simulink model "scd3busMicrogridDroopControlFidelityLevels2Inv"  (R2025b)
settings: Solver=ode15s  StartTime=0.0  StopTime=24  RelTol=1e-3
PreLoadFcn:
  | scd3busMicrogridDroopControlDataFidelityLevels2Inv;
  | 
  | %% Controller variants
  | % Create variant controls for converter controller. Controller has two
  | % different levels of fidelity: Averaged, AveragedPulse, Pulse
  | Averaged = Simulink.VariantExpression;
  | Averaged.Condition = 'fidelity==scd3busMicrogridDroopControl_variants_enum.Low';
  | Pulse = Simulink.VariantExpression;
  | Pulse.Condition = 'fidelity==scd3busMicrogridDroopControl_variants_enum.High';
  | 
  | %% Plant variants
  | % Create variant controls for converter plant. Plant has three different
  | % levels of fidelity.
  | AveragedNonSwitch = Simulink.VariantExpression;
  | AveragedNonSwitch.Condition = 'fidelity==scd3busMicrogridDroopControl_variants_enum.Low';
  | PulseSwitch = Simulink.VariantExpression;
  | PulseSwitch.Condition = 'fidelity==scd3busMicrogridDroopControl_variants_enum.High';
  | 
  | %% Set up variables ready for simulation
  | fidelity = scd3busMicrogridDroopControl_variants_enum.High;
  | Ts = 5e-6;
  | Ts_V = 1e-6;
  | Tsc = 1e-4;
  | Tsc_V = 5e-4;
values from neighbouring files (symbols this model uses):
  consensus_enable = 1    [scd3busMicrogridDroopControlDataFidelityLevels3Inv.m]
  fgrid = 60    [scd3busMicrogridDroopControlDataFidelityLevels.m]    (also in scd3busMicrogridDroopControlDataFidelityLevels3Inv.m)
  Kdroop_fp1 = 0.03/2    (= 0.015)    [scd3busMicrogridDroopControlDataFidelityLevels3Inv.m]
  Kdroop_fp2 = 0.03/2    (= 0.015)    [scd3busMicrogridDroopControlDataFidelityLevels3Inv.m]
  Kdroop_vq1 = 0.05/2    (= 0.025)    [scd3busMicrogridDroopControlDataFidelityLevels3Inv.m]
  Kdroop_vq2 = 0.05/2    (= 0.025)    [scd3busMicrogridDroopControlDataFidelityLevels3Inv.m]
  Ki_vd = 850    [scd3busMicrogridDroopControlDataFidelityLevels.m]    (also in scd3busMicrogridDroopControlDataFidelityLevels3Inv.m)
  Ki_vq = 850    [scd3busMicrogridDroopControlDataFidelityLevels.m]    (also in scd3busMicrogridDroopControlDataFidelityLevels3Inv.m)
  Kp_vd = 0.36    [scd3busMicrogridDroopControlDataFidelityLevels.m]    (also in scd3busMicrogridDroopControlDataFidelityLevels3Inv.m)
  Kp_vq = 0.36    [scd3busMicrogridDroopControlDataFidelityLevels.m]    (also in scd3busMicrogridDroopControlDataFidelityLevels3Inv.m)
  Vdc1 = 1000    [scd3busMicrogridDroopControlDataFidelityLevels.m]    (also in scd3busMicrogridDroopControlDataFidelityLevels3Inv.m)
  Vdc2 = 1000    [scd3busMicrogridDroopControlDataFidelityLevels.m]    (also in scd3busMicrogridDroopControlDataFidelityLevels3Inv.m)
  Vrms = 380    [scd3busMicrogridDroopControlDataFidelityLevels.m]    (also in scd3busMicrogridDroopControlDataFidelityLevels3Inv.m)
undefined symbols (not defined in the file or in its folder): DiscIntNeverNeededParam
libraries: ee_lib x29, nesl_utility x29, fl_lib x17, eeTransforms x4, eeSinusoidalMeasurement x4, slpidlib x4, eePwmGeneratorTwoLevel x2, eePowerMeasurement x2, simulink x2, SignalEditorBlockLib x1
(part 3 of 3)

== system scd3busMicrogridDroopControlFidelityLevels2Inv/Inverter 2/Averaged Inverter ==
  Averaged Inverter : ee_lib/Semiconductors & Converters/Converters/Converter (Three-Phase)  port_option=ee.enum.threePhasePort.expanded  fidelity_option=ee.enum.converters.fidelity.detailed  device_type=ee.enum.converters.switchingdevice.averaged  showThermalPort=false  K=0  Vth=0.5 V  Vgt=1e-3 V  Vgt_off=-1 V  Ih=1 A  Vf=0.8 V  Ron=1.0000e-03 Ohm  Rds=0.001 Ohm  Goff=2.0000e-04 1/Ohm  Eon_scalar=22.86e-3 J  Eoff_scalar=17.14e-3 J  Eoff_natural_commutation=10e-3 J  Voff=300 V  Iout_scalar=600 A  onCurrentMeasDelay=0 s  useCurrentFromPreviousCycle=false  useVoltageFromPreviousCycle=false  diode_param=ee.enum.converters.protectiondiode.nodynamics  diode_Vf=0.8 V  diode_Ron=0.001 Ohm  diode_Goff=1e-5 1/Ohm  diode_C=50 nF  diode_iRM=-235 A  diode_iF=300 A  diode_idot=-50 A/us  diode_trr_param=ee.enum.converters.diodetrr.trr_factor  diode_trr_factor=3  diode_trr=15 us  diode_Qrr=1.5e+3 s*uA  diode_rec_loss_model=ee.enum.diode.reverseRecoveryModel.fixed  diode_ErecVal=0 J  diode_scaleWithIandV=false  diode_ErecMat=zeros(2, 3) J  diode_TjrecVec=[298.15, 398.15] K  diode_IfrecVec=[.1, 1, 10] A  diode_IrecVal=10 A  diode_VrecVal=10 V  diode_tFilter=1 / 1000 / 100 s  thermal_network_parameterization=ee.enum.thermalNetworkTopology.external  Rth=[.08, .5] K/W  Rth_Cauer=[.08, .1, .5] K/W  Rth_Foster=[.08, .14, .22, .16] K/W  thermal_mass_parameterization=ee.enum.thermalNetwork.timeconstant  thermal_mass=[.01, .5] J/K  thermal_mass_Cauer=[.01, .1, .5] J/K  thermal_mass_Foster=[.001, .005, .05, .5] J/K  thermal_time_constant=[.001, .2] s  thermal_time_constant_Cauer=[.001, .1, .2] s  thermal_time_constant_Foster=[7e-05, .0007, .01, .08] s  thermal_mass_initial_temperatures=[25, 25] degC  thermal_mass_initial_temperatures_Cauer=[25, 25, 25] degC  junction_thermal_mass=0.01 J/K  Tvec_initial_Foster=[25, 25, 25, 25] degC  snubber_type=ee.enum.converters.snubber.exclude  Cs=1e-7 F  Rs=0.1 Ohm  Vce_loss=[0, 150, 300] V
      settings: InternalSimscapePortConfiguration="{\"Bottom\":[],\"Left\":[{\"id\":\"G\",\"label\":\"G\",\"type\":\"foundation.electrical.twelve_phase\"},{\"id\":\"a\",\"label\":\"a\",\"type\":\"foundation.electrical.electrical\"},{\"id\":\"b\",\"label\":\"b\",\"type\":\"foundation.electrical.electrical\"},{\"id\":\"c\",\"label\":\"c\",\"type\":\"foundation.electrical.electrical\"}],\"Right\":[{\"id\":\"p\",\"label\":\"+\",\"type\":\"foundation.electrical.electrical\"},{\"id\":\"n\",\"label\":\"-\",\"type\":\"foundation.electrical.electrical\"}],\"Top\":[]}"
  + : PMIOPort  Side=Right
  G : PMIOPort  Port=2  Side=Left
  a : PMIOPort  Port=3  Side=Left
  b : PMIOPort  Port=4  Side=Left
  - : PMIOPort  Port=5  Side=Right
  c : PMIOPort  Port=6  Side=Left
  connections:
  +/RConn1 -- Averaged Inverter/RConn1
  b/RConn1 -- Averaged Inverter/LConn3
  -/RConn1 -- Averaged Inverter/RConn2
  G/RConn1 -- Averaged Inverter/LConn1
  a/RConn1 -- Averaged Inverter/LConn2
  c/RConn1 -- Averaged Inverter/LConn4

== system scd3busMicrogridDroopControlFidelityLevels2Inv/Inverter 2/IGBT Inverter ==
  IGBT Inverter : ee_lib/Semiconductors & Converters/Converters/Converter (Three-Phase)  port_option=ee.enum.threePhasePort.expanded  fidelity_option=ee.enum.converters.fidelity.detailed  device_type=ee.enum.converters.switchingdevice.igbt  showThermalPort=false  K=0  Vth=0.5 V  Vgt=1e-3 V  Vgt_off=-1 V  Ih=1 A  Vf=0.8 V  Ron=1.0000e-03 Ohm  Rds=0.001 Ohm  Goff=2.0000e-04 1/Ohm  Eon_scalar=22.86e-3 J  Eoff_scalar=17.14e-3 J  Eoff_natural_commutation=10e-3 J  Voff=300 V  Iout_scalar=600 A  onCurrentMeasDelay=0 s  useCurrentFromPreviousCycle=false  useVoltageFromPreviousCycle=false  diode_param=ee.enum.converters.protectiondiode.nodynamics  diode_Vf=0.8 V  diode_Ron=0.001 Ohm  diode_Goff=1e-5 1/Ohm  diode_C=50 nF  diode_iRM=-235 A  diode_iF=300 A  diode_idot=-50 A/us  diode_trr_param=ee.enum.converters.diodetrr.trr_factor  diode_trr_factor=3  diode_trr=15 us  diode_Qrr=1.5e+3 s*uA  diode_rec_loss_model=ee.enum.diode.reverseRecoveryModel.fixed  diode_ErecVal=0 J  diode_scaleWithIandV=false  diode_ErecMat=zeros(2, 3) J  diode_TjrecVec=[298.15, 398.15] K  diode_IfrecVec=[.1, 1, 10] A  diode_IrecVal=10 A  diode_VrecVal=10 V  diode_tFilter=1 / 1000 / 100 s  thermal_network_parameterization=ee.enum.thermalNetworkTopology.external  Rth=[.08, .5] K/W  Rth_Cauer=[.08, .1, .5] K/W  Rth_Foster=[.08, .14, .22, .16] K/W  thermal_mass_parameterization=ee.enum.thermalNetwork.timeconstant  thermal_mass=[.01, .5] J/K  thermal_mass_Cauer=[.01, .1, .5] J/K  thermal_mass_Foster=[.001, .005, .05, .5] J/K  thermal_time_constant=[.001, .2] s  thermal_time_constant_Cauer=[.001, .1, .2] s  thermal_time_constant_Foster=[7e-05, .0007, .01, .08] s  thermal_mass_initial_temperatures=[25, 25] degC  thermal_mass_initial_temperatures_Cauer=[25, 25, 25] degC  junction_thermal_mass=0.01 J/K  Tvec_initial_Foster=[25, 25, 25, 25] degC  snubber_type=ee.enum.converters.snubber.exclude  Cs=1e-7 F  Rs=0.1 Ohm  Vce_loss=[0, 150, 300] V
      settings: InternalSimscapePortConfiguration="{\"Bottom\":[],\"Left\":[{\"id\":\"G\",\"label\":\"G\",\"type\":\"foundation.electrical.twelve_phase\"},{\"id\":\"a\",\"label\":\"a\",\"type\":\"foundation.electrical.electrical\"},{\"id\":\"b\",\"label\":\"b\",\"type\":\"foundation.electrical.electrical\"},{\"id\":\"c\",\"label\":\"c\",\"type\":\"foundation.electrical.electrical\"}],\"Right\":[{\"id\":\"p\",\"label\":\"+\",\"type\":\"foundation.electrical.electrical\"},{\"id\":\"n\",\"label\":\"-\",\"type\":\"foundation.electrical.electrical\"}],\"Top\":[]}"
  + : PMIOPort  Side=Right
  G : PMIOPort  Port=2  Side=Left
  a : PMIOPort  Port=3  Side=Left
  b : PMIOPort  Port=4  Side=Left
  - : PMIOPort  Port=5  Side=Right
  c : PMIOPort  Port=6  Side=Left
  connections:
  c/RConn1 -- IGBT Inverter/LConn4
  a/RConn1 -- IGBT Inverter/LConn2
  G/RConn1 -- IGBT Inverter/LConn1
  -/RConn1 -- IGBT Inverter/RConn2
  b/RConn1 -- IGBT Inverter/LConn3
  +/RConn1 -- IGBT Inverter/RConn1

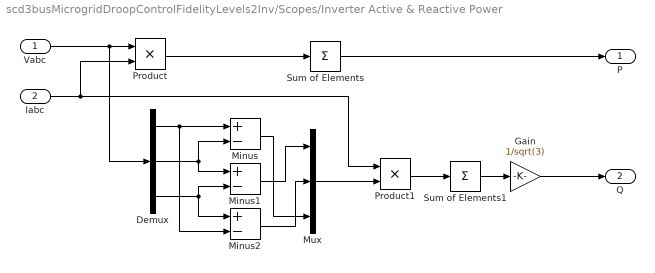
== system scd3busMicrogridDroopControlFidelityLevels2Inv/Scopes/Inverter Active & Reactive Power  ==
  Vabc : Inport
  Iabc : Inport  Port=2
  Demux : Demux  Outputs=3
  Gain : Gain  Gain=1/sqrt(3)
  Minus : Sum  Inputs=+-
  Minus1 : Sum  Inputs=+-
  Minus2 : Sum  Inputs=+-
  Mux : Mux  Inputs=3
  Product : Product
  Product1 : Product
  Sum of Elements : Sum  Inputs=+
  Sum of Elements1 : Sum  Inputs=+
  P : Outport  VectorParamsAs1DForOutWhenUnconnected=off
  Q : Outport  Port=2  VectorParamsAs1DForOutWhenUnconnected=off
  wires:
  Minus/1 -> Mux/3
  Minus2/1 -> Mux/2
  Minus1/1 -> Mux/1
  Gain/1 -> Q/1
  Sum of Elements1/1 -> Gain/1
  Product1/1 -> Sum of Elements1/1
  Mux/1 -> Product1/2
  Demux/3 -> Minus1/2, Minus2/1
  Demux/2 -> Minus/2, Minus1/1
  Demux/1 -> Minus/1, Minus2/2
  Sum of Elements/1 -> P/1
  Product/1 -> Sum of Elements/1
  Iabc/1 -> Product/2, Product1/1
  Vabc/1 -> Product/1, Demux/1

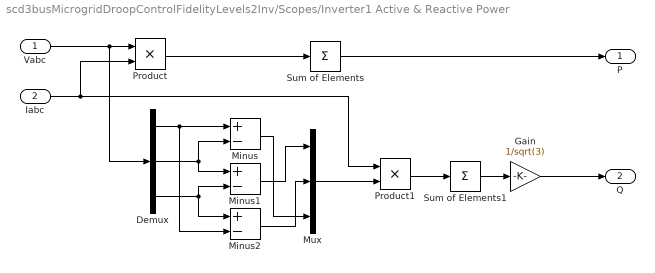
== system scd3busMicrogridDroopControlFidelityLevels2Inv/Scopes/Inverter1 Active & Reactive Power ==
  Vabc : Inport
  Iabc : Inport  Port=2
  Demux : Demux  Outputs=3
  Gain : Gain  Gain=1/sqrt(3)
  Minus : Sum  Inputs=+-
  Minus1 : Sum  Inputs=+-
  Minus2 : Sum  Inputs=+-
  Mux : Mux  Inputs=3
  Product : Product
  Product1 : Product
  Sum of Elements : Sum  Inputs=+
  Sum of Elements1 : Sum  Inputs=+
  P : Outport  VectorParamsAs1DForOutWhenUnconnected=off
  Q : Outport  Port=2  VectorParamsAs1DForOutWhenUnconnected=off
  wires:
  Vabc/1 -> Demux/1, Product/1
  Iabc/1 -> Product1/1, Product/2
  Product/1 -> Sum of Elements/1
  Sum of Elements/1 -> P/1
  Demux/1 -> Minus2/2, Minus/1
  Demux/2 -> Minus1/1, Minus/2
  Demux/3 -> Minus2/1, Minus1/2
  Mux/1 -> Product1/2
  Product1/1 -> Sum of Elements1/1
  Sum of Elements1/1 -> Gain/1
  Gain/1 -> Q/1
  Minus1/1 -> Mux/1
  Minus2/1 -> Mux/2
  Minus/1 -> Mux/3

== system scd3busMicrogridDroopControlFidelityLevels2Inv/Solar1/MPPT Algorithm ==
  I : Inport
  V : Inport  Port=2
  D_init : Constant  Value=0.25
  D_max : Constant  Value=0.4
  D_min : Constant  Value=0.15
  Delta_D : Constant  Value=0.001
  MPPT Algorithm : MATLAB Function  SystemSampleTime=Ts
  Unit Delay : UnitDelay  InitialCondition=0.2  SampleTime=0.01
  Vector Concatenate : Concatenate  NumInputs=4
  duty_cycle : Outport
  wires:
  V/1 -> MPPT Algorithm/2(V)
  Vector Concatenate/1 -> MPPT Algorithm/1(Param)
  D_max/1 -> Vector Concatenate/2
  D_init/1 -> Vector Concatenate/1
  D_min/1 -> Vector Concatenate/3
  MPPT Algorithm/1(D) -> Unit Delay/1
  Delta_D/1 -> Vector Concatenate/4
  I/1 -> MPPT Algorithm/3(I)
  Unit Delay/1 -> duty_cycle/1

== system scd3busMicrogridDroopControlFidelityLevels2Inv/Solar1/Sensing Current ==
  Current Sensor : fl_lib/Electrical/Electrical Sensors/Current Sensor
  PS-Simulink/I : nesl_utility/PS-Simulink Converter  PhysicalDomain=network_engine_domain  SubClassName=ps_output  LeftPortType=input  RightPortType=output  PseudoPeriodic=off  Frequencies=[]  VectorFormat=1-D array  Unit=1  AffineConversion=off
  + : PMIOPort  Side=Left
  - : PMIOPort  Port=2  Side=Right
  I : Outport
  wires:
  PS-Simulink/I/1 -> I/1
  connections:
  -/RConn1 -- Current Sensor/RConn2
  Current Sensor/LConn1 -- +/RConn1
  Current Sensor/RConn1 -- PS-Simulink/I/LConn1

== system scd3busMicrogridDroopControlFidelityLevels2Inv/Solar1/sensing voltage ==
  PS-Simulink Converter : nesl_utility/PS-Simulink Converter  PhysicalDomain=network_engine_domain  SubClassName=ps_output  LeftPortType=input  RightPortType=output  PseudoPeriodic=off  Frequencies=[]  VectorFormat=1-D array  Unit=inherit  AffineConversion=off
  Voltage Sensor : fl_lib/Electrical/Electrical Sensors/Voltage Sensor
  + : PMIOPort  Side=Left
  - : PMIOPort  Port=2  Side=Right
  V : Outport
  wires:
  PS-Simulink Converter/1 -> V/1
  connections:
  Voltage Sensor/LConn1 -- +/RConn1
  Voltage Sensor/RConn2 -- -/RConn1
  Voltage Sensor/RConn1 -- PS-Simulink Converter/LConn1

== system scd3busMicrogridDroopControlFidelityLevels2Inv/Solar2/MPPT Algorithm ==
  I : Inport
  V : Inport  Port=2
  D_init : Constant  Value=0.25
  D_max : Constant  Value=0.4
  D_min : Constant  Value=0.15
  Delta_D : Constant  Value=0.001
  MPPT Algorithm : MATLAB Function  SystemSampleTime=Ts
  Unit Delay : UnitDelay  InitialCondition=0.2  SampleTime=0.01
  Vector Concatenate : Concatenate  NumInputs=4
  duty_cycle : Outport
  wires:
  V/1 -> MPPT Algorithm/2(V)
  Vector Concatenate/1 -> MPPT Algorithm/1(Param)
  D_max/1 -> Vector Concatenate/2
  D_init/1 -> Vector Concatenate/1
  D_min/1 -> Vector Concatenate/3
  MPPT Algorithm/1(D) -> Unit Delay/1
  Delta_D/1 -> Vector Concatenate/4
  I/1 -> MPPT Algorithm/3(I)
  Unit Delay/1 -> duty_cycle/1

== system scd3busMicrogridDroopControlFidelityLevels2Inv/Solar2/Sensing Current ==
  Current Sensor : fl_lib/Electrical/Electrical Sensors/Current Sensor
  PS-Simulink/I : nesl_utility/PS-Simulink Converter  PhysicalDomain=network_engine_domain  SubClassName=ps_output  LeftPortType=input  RightPortType=output  PseudoPeriodic=off  Frequencies=[]  VectorFormat=1-D array  Unit=1  AffineConversion=off
  + : PMIOPort  Side=Left
  - : PMIOPort  Port=2  Side=Right
  I : Outport
  wires:
  PS-Simulink/I/1 -> I/1
  connections:
  -/RConn1 -- Current Sensor/RConn2
  Current Sensor/LConn1 -- +/RConn1
  Current Sensor/RConn1 -- PS-Simulink/I/LConn1

== system scd3busMicrogridDroopControlFidelityLevels2Inv/Solar2/sensing voltage ==
  PS-Simulink Converter : nesl_utility/PS-Simulink Converter  PhysicalDomain=network_engine_domain  SubClassName=ps_output  LeftPortType=input  RightPortType=output  PseudoPeriodic=off  Frequencies=[]  VectorFormat=1-D array  Unit=inherit  AffineConversion=off
  Voltage Sensor : fl_lib/Electrical/Electrical Sensors/Voltage Sensor
  + : PMIOPort  Side=Left
  - : PMIOPort  Port=2  Side=Right
  V : Outport
  wires:
  PS-Simulink Converter/1 -> V/1
  connections:
  Voltage Sensor/LConn1 -- +/RConn1
  Voltage Sensor/RConn2 -- -/RConn1
  Voltage Sensor/RConn1 -- PS-Simulink Converter/LConn1

== matlab function scd3busMicrogridDroopControlFidelityLevels2Inv/Solar1/MPPT Algorithm/MPPT Algorithm ==
  settings: updateMethod=DISCRETE  sampleTime=Ts_DC
  data: Param input; V input; I input; D output
function D = PandO(Param, V, I)

Dinit  = Param(1);
Dmax   = Param(2);
Dmin   = Param(3);
deltaD = Param(4);

persistent Vold Pold Dold;
if isempty(Vold)
    Vold = 0;
    Pold = 0;
    Dold = Dinit;
end

P  = V * I;
dV = V - Vold;
dP = P - Pold;

%% -- fixed: use a dead-band instead of exact zero comparison --
if abs(dP) < 0.5        % ignore changes smaller than 0.5 W (noise)
    D = Dold;           % already at MPP, hold duty cycle

elseif dP < 0
    if dV < 0
        D = Dold - deltaD;
    else
        D = Dold + deltaD;
    end

else                    % dP > 0
    if dV < 0
        D = Dold + deltaD;
    else
        D = Dold - deltaD;
    end
end

%% -- clamp --
D = max(Dmin, min(Dmax, D));

%% -- update persistent state --
Dold = D;
Vold = V;
Pold = P;

== matlab function scd3busMicrogridDroopControlFidelityLevels2Inv/Droop Controller Inverter1/MATLAB Function ==
  data: omega_1 input; d_omega output; omega_2 input; V_1 input; V_2 input; int_w_in input; int_v_in input; Ts input; d_V output; int_w_out output; int_v_out output
function [d_omega, d_V, int_w_out, int_v_out] = ...
         Consensus_Agent1(omega_1, omega_2, V_1, V_2, ...
                          int_w_in, int_v_in, Ts)
%% Gains — tuned for Hz units and visible correction
alpha_w = 50.0;   beta_w = 30.0;   kref_w = 20.0;
alpha_v = 0.30;   beta_v = 0.20;   kref_v = 0.10;

omega_ref = 60.0;   % Hz — confirmed from your freq_mea display
V_ref     = 1.0;    % pu

%% Frequency
e_omega     = omega_1 - omega_ref;
consensus_w = omega_1 - omega_2;
int_w_out   = max(-0.5, min(0.5, int_w_in + Ts * consensus_w));
d_omega     = -alpha_w*consensus_w - beta_w*int_w_out - kref_w*e_omega;
d_omega     = max(-2.0, min(2.0, d_omega));   % wider clamp

%% Voltage
e_V         = V_1 - V_ref;
consensus_v = V_1 - V_2;
int_v_out   = max(-0.20, min(0.20, int_v_in + Ts * consensus_v));
d_V         = -alpha_v*consensus_v - beta_v*int_v_out - kref_v*e_V;
d_V         = max(-0.15, min(0.15, d_V));
end

== matlab function scd3busMicrogridDroopControlFidelityLevels2Inv/Droop Controller Inverter2/MATLAB Function ==
  data: omega_2 input; d_omega output; omega_1 input; V_2 input; V_1 input; int_w_in input; int_v_in input; Ts input; d_V output; int_w_out output; int_v_out output
function [d_omega, d_V, int_w_out, int_v_out] = ...
         Consensus_Agent2(omega_2, omega_1, V_2, V_1, ...
                          int_w_in, int_v_in, Ts)
%% Identical gains to Agent 1
alpha_w = 50.0;   beta_w = 30.0;   kref_w = 20.0;
alpha_v = 0.30;   beta_v = 0.20;   kref_v = 0.10;

omega_ref = 60.0;
V_ref     = 1.0;

%% Frequency
e_omega     = omega_2 - omega_ref;
consensus_w = omega_2 - omega_1;
int_w_out   = max(-0.5, min(0.5, int_w_in + Ts * consensus_w));
d_omega     = -alpha_w*consensus_w - beta_w*int_w_out - kref_w*e_omega;
d_omega     = max(-2.0, min(2.0, d_omega));

%% Voltage
e_V         = V_2 - V_ref;
consensus_v = V_2 - V_1;
int_v_out   = max(-0.20, min(0.20, int_v_in + Ts * consensus_v));
d_V         = -alpha_v*consensus_v - beta_v*int_v_out - kref_v*e_V;
d_V         = max(-0.15, min(0.15, d_V));
end

== matlab function scd3busMicrogridDroopControlFidelityLevels2Inv/Solar2/MPPT Algorithm/MPPT Algorithm ==
  settings: updateMethod=DISCRETE  sampleTime=Ts_DC
  data: Param input; V input; I input; D output
function D = PandO(Param, V, I)

Dinit  = Param(1);
Dmax   = Param(2);
Dmin   = Param(3);
deltaD = Param(4);

persistent Vold Pold Dold;
if isempty(Vold)
    Vold = 0;
    Pold = 0;
    Dold = Dinit;
end

P  = V * I;
dV = V - Vold;
dP = P - Pold;

%% -- fixed: use a dead-band instead of exact zero comparison --
if abs(dP) < 0.5        % ignore changes smaller than 0.5 W (noise)
    D = Dold;           % already at MPP, hold duty cycle

elseif dP < 0
    if dV < 0
        D = Dold - deltaD;
    else
        D = Dold + deltaD;
    end

else                    % dP > 0
    if dV < 0
        D = Dold + deltaD;
    else
        D = Dold - deltaD;
    end
end

%% -- clamp --
D = max(Dmin, min(Dmax, D));

%% -- update persistent state --
Dold = D;
Vold = V;
Pold = P;
